simulink subsystem "Sonares"  (R2023b)
settings: Solver=VariableStepAuto  StartTime=0.0  StopTime=10.0  RelTol=1e-3
libraries: arduinolib x2
settings Model: Creator=marqu  LastModifiedBy=marqu

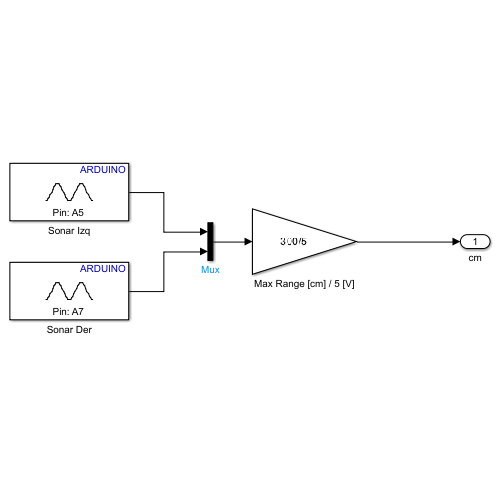
[thumbnail: Simulink's stored preview of the top-level diagram]
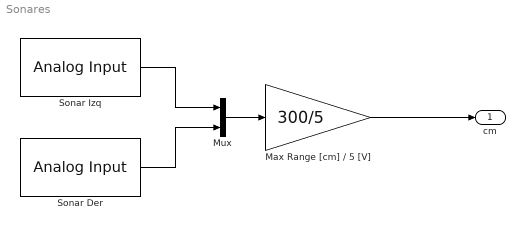
== system Sonares ==
  Max Range [cm] / 5 [V] : Gain  Gain=300/5
  Mux : Mux  Inputs=2
  Sonar Der : arduinolib/Analog Input  pinNumber=7  ReadResultsOnly=off  ConversionTriggerSource=Software  ExternalTriggerType=uint32( 0 )  OutputDataType=uint16  EnableConversionCompleteNotify=off  EnableOuputStatus=off  SampleTime=.1  blockPlatform=arduino
  Sonar Izq : arduinolib/Analog Input  pinNumber=5  ReadResultsOnly=off  ConversionTriggerSource=Software  ExternalTriggerType=uint32( 0 )  OutputDataType=uint16  EnableConversionCompleteNotify=off  EnableOuputStatus=off  SampleTime=.1  blockPlatform=arduino
  cm : Outport
  wires:
  Sonar Der/1 -> Mux/2
  Sonar Izq/1 -> Mux/1
  Mux/1 -> Max Range [cm] / 5 [V]/1
  Max Range [cm] / 5 [V]/1 -> cm/1
